simulink model "testRamp"  (R2024b)
settings: Solver=VariableStepAuto  StartTime=0.0  StopTime=10.0  RelTol=1e-3
PreLoadFcn:
  | m = 10; %mass
  | k = 1e4; %stiffness
  | b = 1e2; %damping
  | F = 10; %input force
  | d2c = 1;
undefined symbols (not defined in the file or in its folder): sampleTime
settings Model: VariantFading=off  Creator=grouleau  LastModifiedBy=grouleau

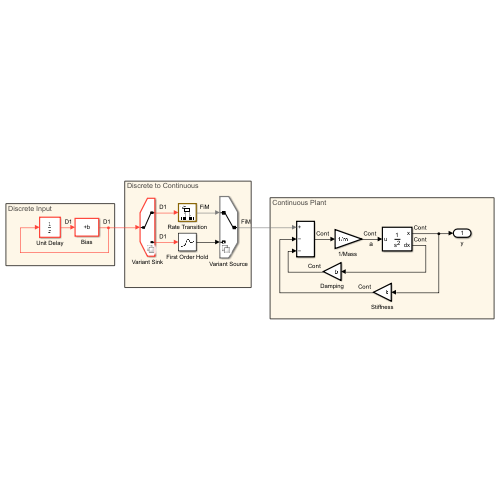
[thumbnail: Simulink's stored preview of the top-level diagram]
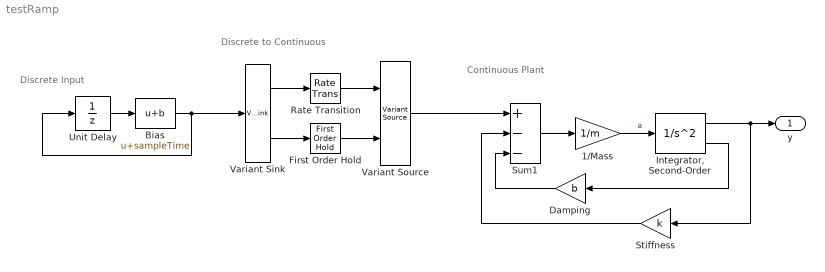
== system testRamp ==
  note: Discrete to Continuous
  note: Discrete Input
  note: Continuous Plant
  "1/Mass " : Gain  Gain=1/m  SaturateOnIntegerOverflow=on  OutDataTypeStr=Inherit: Same as input  ParamDataTypeStr=Inherit: Same as input
  Bias : Bias  Bias=sampleTime  SaturateOnIntegerOverflow=off
  Damping : Gain  Gain=b  SaturateOnIntegerOverflow=on  OutDataTypeStr=Inherit: Same as input  ParamDataTypeStr=Inherit: Same as input
  First Order Hold : FirstOrderHold  ErrorTolerance=inf
  "Integrator, Second-Order" : SecondOrderIntegrator
  Rate Transition : RateTransition
  Stiffness : Gain  Gain=k  SaturateOnIntegerOverflow=on  OutDataTypeStr=Inherit: Same as input  ParamDataTypeStr=Inherit: Same as input
  Sum1 : Sum  Inputs=+--  InputSameDT=on  SaturateOnIntegerOverflow=on  OutDataTypeStr=Inherit: Same as first input
  Unit Delay : UnitDelay  SampleTime=sampleTime  HasFrameUpgradeWarning=on
  Variant Sink : VariantSink
  Variant Source : VariantSource
  y : Outport
  wires:
  Stiffness/1 -> Sum1/2
  Damping/1 -> Sum1/3
  "Integrator, Second-Order"/1 -> y/1, Stiffness/1
  Sum1/1 -> "1/Mass "/1
  "1/Mass "/1 -> "Integrator, Second-Order"/1  "a"
  "Integrator, Second-Order"/2 -> Damping/1
  Variant Source/1 -> Sum1/1
  Variant Sink/1 -> Rate Transition/1
  Rate Transition/1 -> Variant Source/1
  First Order Hold/1 -> Variant Source/2
  Variant Sink/2 -> First Order Hold/1
  Bias/1 -> Variant Sink/1, Unit Delay/1
  Unit Delay/1 -> Bias/1
